simulink model "simulink_random_error"  (R2016b)
settings: Solver=FixedStepAuto  StartTime=0.0  StopTime=Tend  FixedStep=hp  RelTol=1e-3
undefined symbols (not defined in the file): error_probability, Sm
settings Model: SimulationMode=accelerator  SnapshotInterval=2  Creator=juan  LastModifiedBy=jvalencia

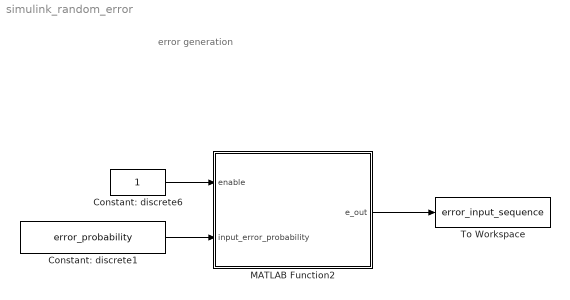
== system simulink_random_error ==
  note: error generation
  Constant: discrete1 : Constant  Value=error_probability  SampleTime=Sm
  Constant: discrete6 : Constant  SampleTime=Sm
  MATLAB Function2 : MATLAB Function  TreatAsAtomicUnit=on  SystemSampleTime=Sm
  To Workspace : ToWorkspace  VariableName=error_input_sequence  SaveFormat=Timeseries  SampleTime=Sm
  wires:
  Constant: discrete1/1 -> MATLAB Function2/2(input_error_probability)
  MATLAB Function2/1(e_out) -> To Workspace/1
  Constant: discrete6/1 -> MATLAB Function2/1(enable)

== matlab function simulink_random_error/MATLAB Function2 ==
  data: e_out output; enable input; input_error_probability input
function e_out = error_generation(enable, input_error_probability)

persistent counter;
if (isempty(counter)) %It does not already exist
counter = 1; % initialize with 1
end

%% test sequence: c1 since there are no errors
sequence = 0; 

if ( counter == length(sequence) )
    counter = 1;
else
    counter = counter + 1;
end

e = sequence(counter);


%% test random error
error_probability = input_error_probability;

temp = unifrnd(0,1);
if (temp > (1-error_probability))
    e = 1;
else
    e = 0;
end


%% enable error injection in the simulation
if enable == 1
    e_out = e;
else
    e_out = 0;
end
